simulink model "Simulink"  (R2021a)
settings: Solver=ode5  StartTime=0.0  StopTime=10  FixedStep=0.001  RelTol=1e-3
values from neighbouring files (symbols this model uses):
  A = [0 0 0 1;0 1446.9 213.6 -57.9;0 1 0 0;0 -126.3 -12.8 5.1]    [1_DiseñoRegulador_Seguidor_Discreto.m]    (also in Control_Seguimiento_Integrador_MATLAB.m = [0,1,0,0;0,-0.221772837618740,0.450086090591265,-0.661704776; Controlador.m = [0 1 0 0;0 -6.109*10^(-08)   2.828*10^(-5)  -7.749*10^(-6);0; Leo_Controlador.m = [0,1,0,0;0,-18.1491205715699,-0.241940259070541,-0.001617883; funcmotor.m = [0 1 0 0;0 par(1) par(2) par(3);0 0 0 1;0 par(4) par(5) par()
  B = [0;-122.6;0;10.7]    [1_DiseñoRegulador_Seguidor_Discreto.m]    (also in Control_Seguimiento_Integrador_MATLAB.m = [0;1.02819574469726;0;2.93672730148517]; Controlador.m = [0;-2.126*10^(-8);0;-293]; Leo_Controlador.m = [0;3.24704785577389;0;142.313463961677]; funcmotor.m = [0;par(7);0;par(8)])
  C = [1 0 0 0]    [1_DiseñoRegulador_Seguidor_Discreto.m]    (also in Control_Seguimiento_Integrador_MATLAB.m = [0 0 1 0]; Controlador.m = [0 0 1 0]; Leo_Controlador.m = [1 0 0 0;0 1 0 0;0 0 1 0; 0 0 0 1]; funcmotor.m = [0 0 1 0;1 0 0 0])
  D = [0]    [1_DiseñoRegulador_Seguidor_Discreto.m]    (also in Control_Seguimiento_Integrador_MATLAB.m; Controlador.m; Leo_Controlador.m = [0;0;0;0]; funcmotor.m = zeros(2,1))
  k1 = Ka(1)    [1_DiseñoRegulador_Seguidor_Discreto.m]    (also in Controlador.m = -2.8342e-06; Leo_Controlador.m = K(1))
  k2 = Ka(2)    [1_DiseñoRegulador_Seguidor_Discreto.m]    (also in Controlador.m = -1925900; Leo_Controlador.m = K(2))
  k3 = Ka(3)    [1_DiseñoRegulador_Seguidor_Discreto.m]    (also in Controlador.m = -18.7082; Leo_Controlador.m = K(3))
  k4 = Ka(4)    [1_DiseñoRegulador_Seguidor_Discreto.m]    (also in Controlador.m = -0.1767; Leo_Controlador.m = K(4))
settings Model: Creator=Usuario  LastModifiedBy=Sinso

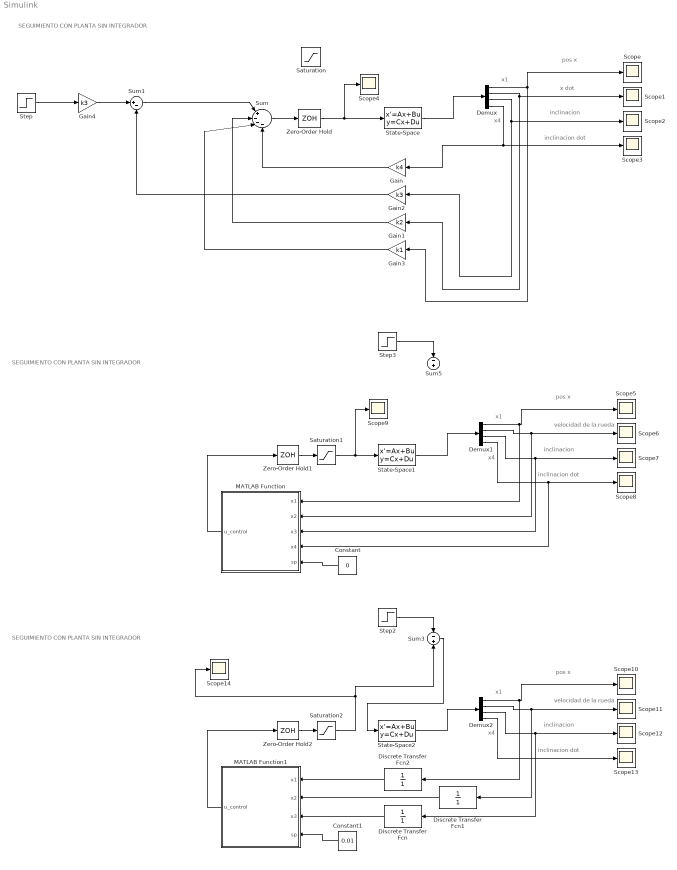
== system Simulink ==
  note: inclinacion dot
  note: inclinacion
  note: x dot
  note: pos x
  note: SEGUIMIENTO CON PLANTA SIN INTEGRADOR
  note: x4
  note: x1
  note: inclinacion
  note: inclinacion dot
  note: pos x
  note: SEGUIMIENTO CON PLANTA SIN INTEGRADOR
  note: x4
  note: x1
  note: velocidad de la rueda
  note: velocidad de la rueda
  note: inclinacion dot
  note: x1
  note: x4
  note: SEGUIMIENTO CON PLANTA SIN INTEGRADOR
  note: pos x
  note: inclinacion
  Constant : Constant  Value=0
  Constant1 : Constant  Value=0.01
  Demux : Demux
  Demux1 : Demux
  Demux2 : Demux
  Discrete Transfer Fcn : DiscreteTransferFcn  Denominator=[1]  SampleTime=0.001
  Discrete Transfer Fcn1 : DiscreteTransferFcn  Denominator=[1]  SampleTime=0.001
  Discrete Transfer Fcn2 : DiscreteTransferFcn  Denominator=[1]  SampleTime=0.001
  Gain : Gain  Gain=k4
  Gain1 : Gain  Gain=k2
  Gain2 : Gain  Gain=k3
  Gain3 : Gain  Gain=k1
  Gain4 : Gain  Gain=k3
  MATLAB Function : MATLAB Function  TreatAsAtomicUnit=on
  MATLAB Function1 : MATLAB Function  TreatAsAtomicUnit=on  SystemSampleTime=0.001
  Saturation : Saturate  UpperLimit=5  LowerLimit=-5
  Saturation1 : Saturate  UpperLimit=5  LowerLimit=-5
  Saturation2 : Saturate  UpperLimit=5  LowerLimit=-5
  Scope{,1..14} (15 alike) : Scope
  State-Space : StateSpace  A=A  B=B  C=C  D=D  InitialCondition=0  ParameterTunability=Optimized
  State-Space1 : StateSpace  A=A  B=B  C=C  D=D  InitialCondition=0  ParameterTunability=Optimized
  State-Space2 : StateSpace  A=A  B=B  C=C  D=D  InitialCondition=0  ParameterTunability=Optimized
  Step : Step  After=0  SampleTime=0
  Step2 : Step  Time=2  After=0  SampleTime=0
  Step3 : Step  Time=2  After=0  SampleTime=0
  Sum : Sum  Inputs=|+---
  Sum1 : Sum  Inputs=|+-
  Sum3 : Sum  Inputs=-+
  Sum5 : Sum  Inputs=-+
  Zero-Order Hold : ZeroOrderHold  SampleTime=0.005
  Zero-Order Hold1 : ZeroOrderHold  SampleTime=0.005
  Zero-Order Hold2 : ZeroOrderHold  SampleTime=0.001
  wires:
  Sum/1 -> Zero-Order Hold/1
  Gain/1 -> Sum/4
  Gain2/1 -> Sum1/2
  Gain1/1 -> Sum/2
  Demux/4 -> Scope3/1, Gain/1
  Demux/3 -> Gain2/1, Scope2/1
  Demux/2 -> Scope1/1, Gain1/1
  Gain4/1 -> Sum1/1
  Step/1 -> Gain4/1
  Demux/1 -> Gain3/1, Scope/1
  Gain3/1 -> Sum/3
  Sum1/1 -> Sum/1
  State-Space/1 -> Demux/1
  Demux1/4 -> MATLAB Function/4(x4), Scope8/1
  Saturation1/1 -> State-Space1/1, Scope9/1
  Demux1/2 -> MATLAB Function/2(x2), Scope6/1
  State-Space1/1 -> Demux1/1
  Demux1/1 -> MATLAB Function/1(x1), Scope5/1
  Zero-Order Hold1/1 -> Saturation1/1
  Demux1/3 -> Scope7/1, MATLAB Function/3(x3)
  Step3/1 -> Sum5/1
  MATLAB Function/1(u_control) -> Zero-Order Hold1/1
  Constant/1 -> MATLAB Function/5(sp)
  Step2/1 -> Sum3/1
  Demux2/3 -> Scope12/1, Discrete Transfer Fcn/1
  Sum3/1 -> State-Space2/1
  Demux2/1 -> Discrete Transfer Fcn2/1, Scope10/1
  Zero-Order Hold2/1 -> Saturation2/1
  State-Space2/1 -> Demux2/1
  Demux2/2 -> Discrete Transfer Fcn1/1, Scope11/1
  Demux2/4 -> Scope13/1
  MATLAB Function1/1(u_control) -> Zero-Order Hold2/1
  Saturation2/1 -> Scope14/1, Sum3/2
  Constant1/1 -> MATLAB Function1/4(sp)
  Zero-Order Hold/1 -> Scope4/1, State-Space/1
  Discrete Transfer Fcn2/1 -> MATLAB Function1/1(x1)
  Discrete Transfer Fcn1/1 -> MATLAB Function1/2(x2)
  Discrete Transfer Fcn/1 -> MATLAB Function1/3(x3)

== matlab function Simulink/MATLAB Function1 ==
  settings: updateMethod=DISCRETE
  data: x1 input; u_control output; x2 input; x3 input; sp input
function u_control = fcn(x1,x2,x3,sp)

k1=-2.8342*10^(-6);
k2=-1.9259*10^(6);
k3=-18.7082;
k4=-0.1767;
g1=k3;
T=0.001;

persistent x3_ant;

if isempty(x3_ant)
    x3_ant=0;
end

x4=(x3-x3_ant)/T;

u_control=g1*sp-(k1*x1+k2*x2+k3*x3+k4*x4);

x3_ant=x3;

== matlab function Simulink/MATLAB Function ==
  data: x1 input; u_control output; x2 input; x3 input; x4 input; sp input
function u_control = fcn(x1,x2,x3,x4,sp)

k1=-2.8342*10^(-6);
k2=-1.9259*10^(6);
k3=-18.7082;
k4=-0.1767;
g1=k3;

% persistent e_1;
% persistent pos_medida_1;

% if isempty(e_1)
%     e_1=0;
%     pos_medida_1=0;
% end

u_control=g1*sp-(k1*x1+k2*x2+k3*x3+k4*x4);

% e_1=e;
% pos_medida_1=pos_medida;
